simulink library "cstm_interfaces_lib"  (R2020a)
settings: Solver=VariableStepAuto  StartTime=0.0  StopTime=10.0  RelTol=1e-3
settings Model: Creator=niekl  LastModifiedBy=niekl

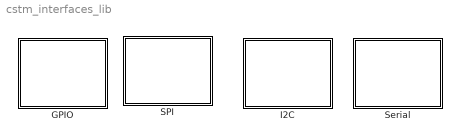
== system cstm_interfaces_lib ==
  GPIO : Subsystem
  I2C : Subsystem
  SPI : Subsystem
  Serial : Subsystem

== system cstm_interfaces_lib/GPIO ==
  cstm_GPIO_read : Subsystem  SystemSampleTime=inf  mask{port=0, OutDataTypeStr=boolean, SampleTime=-1}
      mask prompts: port "GPIO chip number"; OutDataTypeStr "Simulink:blkprm_prompts:OUTPUT_UNIFIEDDATATYPE"; SampleTime "Simulink:blkprm_prompts:AllBlksSampleTime"
      mask TypeOptions OutDataTypeStr: Cast To Boolean/OutDataTypeStr
      mask TypeOptions SampleTime: Val/SampleTime
      mask DialogControl OutDataTypeStr Prompt: Output data type:
      mask DialogControl SampleTime Prompt: Sample time (-1 for inherited):
      mask Display:
      | disp('cstm GPIO Read')
      | port_label('output', 1, 'Value')
  cstm_GPIO_write : Subsystem  mask{port=0, OutDataTypeStr=Inherit: auto, SampleTime=-1}
      mask prompts: port "GPIO chip number"; OutDataTypeStr "Simulink:blkprm_prompts:UNIFIEDDATATYPE"; SampleTime "Simulink:blkprm_prompts:AllBlksSampleTime"
      mask TypeOptions OutDataTypeStr: Val/OutDataTypeStr
      mask TypeOptions SampleTime: Val/SampleTime
      mask DialogControl OutDataTypeStr Prompt: Data type:
      mask DialogControl SampleTime Prompt: Sample time (-1 for inherited):
      mask Display:
      | disp('cstm GPIO Write')
      | port_label('input', 1, 'Value')

== system cstm_interfaces_lib/I2C ==
  cstm_I2C_Read : Subsystem  mask{ADAPTERNUMBER=0, ADDRESS=0, BYTEORDERSTRING=BigEndian, ENABLEREG=on, SLAVEREG=0, OutDataTypeStr=uint8, MESSAGESIZE=1, SENDNACKSTRING=on, REMOVESTOPSTRING=on, OUTERROR=off, BYTEORDER=0, SENDREGISTER=1, SENDNACK=1, REMOVESTOP=1}
      mask prompts: ADAPTERNUMBER "Adapter number:"; ADDRESS "Slave address:"; BYTEORDERSTRING "Slave byte order:"; ENABLEREG "Enable register access"; SLAVEREG "Slave register address:"; OutDataTypeStr "Simulink:blkprm_prompts:OUTPUT_UNIFIEDDATATYPE"; MESSAGESIZE "Data size:"; SENDNACKSTRING "Send NACK at end of data transfer"; REMOVESTOPSTRING "Remove stop bit at the end of data transfer"; OUTERROR "Output error status"; BYTEORDER "byte order translate"; SENDREGISTER "slave register address translate"; SENDNACK "send nack translate"; REMOVESTOP "remove stop bit translate"
      mask init:
      | enab = get_param(gcb,'OUTERROR');
      | 
      | % Set the 'MaskVisibilities' property for each parameters
      | if strcmp(enab,'on')
      |     if strcmp(get_param([gcb '/ErrorMessage'],'BlockType'), 'Display')
      |         replace_block(gcb, 'FollowLinks', 'on', 'Name', 'ErrorMessage', 'Outport', 'noprompt')
      |     end
      | else
      |     if strcmp(get_param([gcb '/ErrorMessage'],'BlockType'), 'Outport')
      |         replace_block(gcb, 'FollowLinks', 'on', 'Name', 'ErrorMessage', 'Display', 'noprompt')
      |     end
      | end
      mask TypeOptions BYTEORDERSTRING: BigEndian | LittleEndian
      mask Callback BYTEORDERSTRING:
      | if(strcmp(get_param(gcb,'BYTEORDERSTRING'),'BigEndian'))
      |     set_param(gcb, 'BYTEORDER', '0');
      | else
      |     set_param(gcb, 'BYTEORDER', '1');
      | end
      mask Callback ENABLEREG:
      | % Control parameter visiblity
      | 
      | % unchecked = 'off'
      | % checked = 'on'
      | enab = get_param(gcb,'ENABLEREG');
      | 
      | % Set the 'MaskVisibilities' property for each parameters
      | if strcmp(enab,'on')
      |     set_param(gcb, 'SENDREGISTER', '1');
      |     set_param(gcb,'MaskVisibilities',{'on','on','on','on','on','on','on','off','off','on','off','off','off','off'});
      | else
      |     set_param(gcb, 'SENDREGISTER', '0');
      |     set_param(gcb,'MaskVisibilities',{'on','on','on','on','off','on','on','on','on','on','off','off','off','off'});
      | end
      | 
      | % Note that the value of the bias is not handled here.
      | % See the Initialization tab
      mask TypeOptions OutDataTypeStr: Data Type Conversion/OutDataTypeStr
      mask Callback SENDNACKSTRING:
      | if(strcmp(get_param(gcb,'SENDNACKSTRING'),'off'))
      |     set_param(gcb, 'SENDNACK', '0');
      | else
      |     set_param(gcb, 'SENDNACK', '1');
      | end
      mask Callback REMOVESTOPSTRING:
      | if(strcmp(get_param(gcb,'REMOVESTOPSTRING'),'off'))
      |     set_param(gcb, 'REMOVESTOP', '0');
      | else
      |     set_param(gcb, 'REMOVESTOP', '1');
      | end
      mask DialogControl OutDataTypeStr Prompt: Output data type:
      mask DialogControl Container3 Prompt: hidden parameters for translation
      mask Display:
      | disp('cstm I2C Write')
      | port_label('output', 1, 'Message out')
      | 
      | if strcmp(get_param(gcb,'OUTERROR'),'on')
      |     port_label('output', 2, 'Error out')
      | end
  cstm_I2C_Write : Subsystem  mask{ADAPTERNUMBER=0, ADDRESS=0, BYTEORDERSTRING=BigEndian, ENABLEREG=on, SLAVEREG=0, SENDNACKSTRING=off, REMOVESTOPSTRING=off, OUTERROR=off, BYTEORDER=0, SENDREGISTER=1, SENDNACK=0, REMOVESTOP=0}
      mask prompts: ADAPTERNUMBER "Adapter number:"; ADDRESS "Slave address:"; BYTEORDERSTRING "Slave byte order:"; ENABLEREG "Enable register access"; SLAVEREG "Slave register address:"; SENDNACKSTRING "Send NACK at end of data transfer"; REMOVESTOPSTRING "Remove stop bit at the end of data transfer"; OUTERROR "Output error status"; BYTEORDER "byte order translate"; SENDREGISTER "slave register address translate"; SENDNACK "send nack translate"; REMOVESTOP "remove stop bit translate"
      mask init: same as cstm_interfaces_lib/I2C/cstm_I2C_Read
      mask TypeOptions BYTEORDERSTRING: BigEndian | LittleEndian
      mask Callback BYTEORDERSTRING:
      | if(strcmp(get_param(gcb,'BYTEORDERSTRING'),'BigEndian'))
      |     set_param(gcb, 'BYTEORDER', '0');
      | else
      |     set_param(gcb, 'BYTEORDER', '1');
      | end
      mask Callback ENABLEREG:
      | % Control parameter visiblity
      | 
      | % unchecked = 'off'
      | % checked = 'on'
      | enab = get_param(gcb,'ENABLEREG');
      | 
      | % Set the 'MaskVisibilities' property for each parameters
      | if strcmp(enab,'on')
      |     set_param(gcb, 'SENDREGISTER', '1');
      |     set_param(gcb,'MaskVisibilities',{'on','on','on','on','on','off','off','on','off','off','off','off'});
      | else
      |     set_param(gcb, 'SENDREGISTER', '0');
      |     set_param(gcb,'MaskVisibilities',{'on','on','on','on','off','on','on','on','off','off','off','off'});
      | end
      | 
      | % Note that the value of the bias is not handled here.
      | % See the Initialization tab
      mask Callback SENDNACKSTRING:
      | if(strcmp(get_param(gcb,'SENDNACKSTRING'),'off'))
      |     set_param(gcb, 'SENDNACK', '0');
      | else
      |     set_param(gcb, 'SENDNACK', '1');
      | end
      mask Callback REMOVESTOPSTRING:
      | if(strcmp(get_param(gcb,'REMOVESTOPSTRING'),'off'))
      |     set_param(gcb, 'REMOVESTOP', '0');
      | else
      |     set_param(gcb, 'REMOVESTOP', '1');
      | end
      mask DialogControl Container3 Prompt: hidden parameters for translation
      mask Display:
      | disp('cstm I2C Write')
      | port_label('input', 1, 'Message in')
      | 
      | if strcmp(get_param(gcb,'OUTERROR'),'on')
      |     port_label('output', 1, 'ErrorOut')
      | end

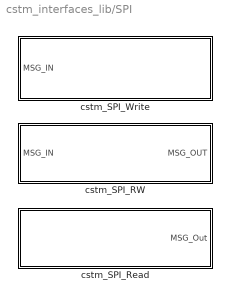
== system cstm_interfaces_lib/SPI ==
  cstm_SPI_RW : Subsystem  mask{Device=0, SlaveSelect=0, SelectedMode=0, RegisterAddress=0, DataLength=1, OutDataTypeStr_in=int8, OutDataTypeStr_out=int8, Sample=-1}
      mask prompts: Device "SPI device:"; SlaveSelect "SPI Slave Select:"; SelectedMode "Mode (Clock polarity and phase):"; RegisterAddress "Register address (-1 for none):"; DataLength "Data length (excluding register):"; OutDataTypeStr_in "Input data type:"; OutDataTypeStr_out "Simulink:blkprm_prompts:OUTPUT_UNIFIEDDATATYPE"; Sample "Sample time (-1 for inherited):"
      mask TypeOptions SelectedMode: 0 | 1 | 2 | 3
      mask DialogControl Control2 Prompt: Mode flag expects a value from 0 to 3: 1 sets phase flag, 2 sets clock polarity flag, and 3 sets both.
      mask DialogControl Control3 Prompt: Data can be read from a register. If this is not desired, set the Register address to -1.
      mask DialogControl Control4 Prompt: Data length expects a positive integer representing the amount of bytes to read. This number is the amount excluding the register address
      mask DialogControl Control6 Prompt: Input data expects a [Nx1] array
      mask DialogControl Control5 Prompt: Output data is a [Nx1] array
      mask DialogControl OutDataTypeStr_out Prompt: Output data type:
      mask Display:
      | disp('cstm SPI Write')
      | port_label('input', 1, 'MessageIn')
      | port_label('output', 1, 'MessageOut')
  cstm_SPI_Read : Subsystem  mask{Device=0, SlaveSelect=0, SelectedMode=0, RegisterAddress=0, DataLength=1, OutDataTypeStr_out=uint8, Sample=-1}
      mask prompts: Device "SPI device:"; SlaveSelect "SPI Slave Select:"; SelectedMode "Mode (Clock polarity and phase):"; RegisterAddress "Register address (-1 for none):"; DataLength "Data length (excluding register):"; OutDataTypeStr_out "Simulink:blkprm_prompts:OUTPUT_UNIFIEDDATATYPE"; Sample "Sample time (-1 for inherited):"
      mask TypeOptions SelectedMode: 0 | 1 | 2 | 3
      mask TypeOptions OutDataTypeStr_out: OutputCastTo/OutDataTypeStr
      mask DialogControl DescTextVar Prompt: Read and write data simultaniously using SPI with an optional register address
      mask DialogControl Control2 Prompt: Mode flag expects a value from 0 to 3: 1 sets phase flag, 2 sets clock polarity flag, and 3 sets both.
      mask DialogControl Control3 Prompt: Data can be read from a register. If this is not desired, set the Register address to -1.
      mask DialogControl Control4 Prompt: Data length expects a positive integer representing the amount of bytes to read and write. This number is the amount excluding the register address
      mask DialogControl Control5 Prompt: Output data is a [Nx1] array
      mask DialogControl OutDataTypeStr_out Prompt: Output data type:
      mask Display:
      | disp('cstm SPI Write')
      | port_label('output', 1, 'MessageOut')
  cstm_SPI_Write : Subsystem  mask{Device=0, SlaveSelect=0, SelectedMode=0, RegisterAddress=0, OutDataTypeStr_out=Inherit: auto, Sample=-1}
      mask prompts: Device "SPI device:"; SlaveSelect "SPI Slave Select:"; SelectedMode "Mode (Clock polarity and phase):"; RegisterAddress "Register address (-1 for none):"; OutDataTypeStr_out "Input data type:"; Sample "Sample time (-1 for inherited):"
      mask TypeOptions SelectedMode: 0 | 1 | 2 | 3
      mask TypeOptions OutDataTypeStr_out: MSG_IN/OutDataTypeStr
      mask DialogControl DescTextVar Prompt: Write data using SPI
      mask DialogControl Control4 Prompt: Mode flag expects a value from 0 to 3: 1 sets phase flag, 2 sets clock polarity flag, and 3 sets both.
      mask DialogControl Control2 Prompt: Data can be written to a register. If this is not desired, set the Register address to -1.
      mask DialogControl Control3 Prompt: Input data expects a [Nx1] array
      mask Display:
      | disp('cstm SPI Write')
      | port_label('input', 1, 'MessageIn')

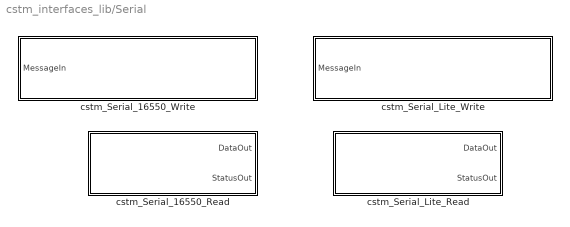
== system cstm_interfaces_lib/Serial ==
  cstm_Serial_16550_Read : Subsystem  mask{PORT=0, BAUDRATE=115200, PARITYSTRING=None, STOPBITS=1, DATALENGTH=1, DATATYPE=int8, SampleTime=-1, BAUDRATESS=0, PARITY=0}
      mask prompts: PORT "Port (ttyS<x>):"; BAUDRATE "Baudrate (in bits/s):"; PARITYSTRING "Parity:"; STOPBITS "Stop bits"; DATALENGTH "Data length (N):"; DATATYPE "Output data type:"; SampleTime "Simulink:blkprm_prompts:AllBlksSampleTime"; BAUDRATESS "baudrate translate"; PARITY "parity translate"
      mask TypeOptions BAUDRATE: 0 | 50 | 75 | 110 | 134 | 150 | 200 | 300 | 600 | 1200 | 1800 | 2400 | 4800 | 9600 | 19200 | 38400 | 57600 | 115200 | 230400
      mask Callback BAUDRATE:
      | % baud = get_param(gcb, 'BAUDRATESTRING')
      | %
      | % switch(baud)
      | %     case '0'
      | %         set_param(gcb,'BAUDRATE','0');
      | %     case '50'
      | %         set_param(gcb,'BAUDRATE','50');
      | %     case '75'
      | %         set_param(gcb,'BAUDRATE','75');
      | %     case '110'
      | %         set_param(gcb,'BAUDRATE','110');
      | %     case '134'
      | %         set_param(gcb,'BAUDRATE','134');
      | %     case '150'
      | %         set_param(gcb,'BAUDRATE','150');
      | %     case '200'
      | %         set_param(gcb,'BAUDRATE','200');
      | %     case '300'
      | %         set_param(gcb,'BAUDRATE','300');
      | %     case '600'
      | %         set_param(gcb,'BAUDRATE','600');
      | %     case '1200'
      | %         set_param(gcb,'BAUDRATE','1200');
      | %     case '0'
      | %         set_param(gcb,'BAUDRATE','1800');
      | %     case '0'
      | %         set_param(gcb,'BAUDRATE','2400');
      | %     case '0'
      | %         set_param(gcb,'BAUDRATE','4800');
      | %     case '0'
      | %         set_param(gcb,'BAUDRATE','9600');
      | %     case '0'
      | %         set_param(gcb,'BAUDRATE','19200');
      | %     case '0'
      | %         set_param(gcb,'BAUDRATE','38400');
      | %     case '0'
      | %         set_param(gcb,'BAUDRATE','57600');
      | %     case '0'
      | %         set_param(gcb,'BAUDRATE','115200');
      | %     case '0'
      | %         set_param(gcb,'BAUDRATE','230400');
      | % end
      mask TypeOptions PARITYSTRING: None | Even | Odd
      mask Callback PARITYSTRING:
      | if(strcmp(get_param(gcb, 'PARITYSTRING'),'none'))
      |     set_param(gcb,'PARITY','0');
      | end
      | if(strcmp(get_param(gcb, 'PARITYSTRING'),'Even'))
      |     set_param(gcb,'PARITY','1');
      | end
      | if(strcmp(get_param(gcb, 'PARITYSTRING'),'Odd'))
      |     set_param(gcb,'PARITY','2');
      | end
      mask TypeOptions STOPBITS: 1 | 2
      mask Callback DATALENGTH:
      | %ph = get_param(gcb,'PortHandles');
      | %length = get_param(gcb, 'DATALENGTH');
      | %set_param([gcb '/DataOut'],'CompiledPortWidths',length);
      mask TypeOptions SampleTime: Data Type Conversion/SampleTime
      mask DialogControl Control2 Prompt: The output: "Message out" is an array of size [Nx1]. Any data presented to UART16550 will be received, upto N bytes (max 256).
      mask DialogControl Control3 Prompt: The output: "Status out" is a [1x1] variable with the amount of read bytes.
      mask DialogControl SampleTime Prompt: Sample time (-1 for inherited):
      mask DialogControl Container3 Prompt: hidden
      mask Display:
      | disp('cstm Serial 16550 Read')
      | port_label('output', 1, 'Message out')
      | port_label('output', 2, 'Status out')
  cstm_Serial_16550_Write : Subsystem  mask{PORT=0, BAUDRATE=0, PARITYSTRING=None, STOPBITS=1, PARITY=0}
      mask prompts: PORT "Port (ttyS<x>):"; BAUDRATE "Baudrate (in bits/s):"; PARITYSTRING "Parity:"; STOPBITS "Stop bits"; PARITY "parity translate"
      mask TypeOptions BAUDRATE: 0 | 50 | 75 | 110 | 134 | 150 | 200 | 300 | 600 | 1200 | 1800 | 2400 | 4800 | 9600 | 19200 | 38400 | 57600 | 115200 | 230400
      mask TypeOptions PARITYSTRING: None | Even | Odd
      mask Callback PARITYSTRING:
      | if(strcmp(get_param(gcb, 'PARITYSTRING'),'none'))
      |     set_param(gcb,'PARITY','0');
      | end
      | if(strcmp(get_param(gcb, 'PARITYSTRING'),'Even'))
      |     set_param(gcb,'PARITY','1');
      | end
      | if(strcmp(get_param(gcb, 'PARITYSTRING'),'Odd'))
      |     set_param(gcb,'PARITY','2');
      | end
      mask TypeOptions STOPBITS: 1 | 2
      mask DialogControl Control2 Prompt: The input is an array of size [Nx1]. Any data presented to UART16550 will be transmitted.
      mask Display:
      | disp('cstm Serial 16550 Write')
      | port_label('input', 1, 'Message in')
  cstm_Serial_Lite_Read : Subsystem  mask{PORT=0, DATALENGTH=0, DATATYPE=int8, SampleTime=-1}
      mask prompts: PORT "Port (ttyUL<x>):"; DATALENGTH "Data length (N):"; DATATYPE "Output data type:"; SampleTime "Simulink:blkprm_prompts:AllBlksSampleTime"
      mask TypeOptions SampleTime: Data Type Conversion/SampleTime
      mask DialogControl DescTextVar Prompt: UARTlite Read accepts only the port as parameter, the device has been pre-configured and cannot be configured in the user space. Contact the SoC developer for details of the UARTlite device in use.
      mask DialogControl Control2 Prompt: The output: "Message out" is an array of size [Nx1]. Any data presented to UARTlite will be received, upto N bytes (max 256).
      mask DialogControl Control2_copy Prompt: The output: "Status out" is a [1x1] variable with the amount of read bytes.
      mask DialogControl SampleTime Prompt: Sample time (-1 for inherited):
      mask Display:
      | disp('cstm Serial Lite Read')
      | port_label('output', 1, 'Message out')
      | port_label('output', 2, 'Status out')
  cstm_Serial_Lite_Write : Subsystem  mask{PORT=0}
      mask prompts: PORT "Port (ttyUL<x>):"
      mask DialogControl DescTextVar Prompt: UARTlite Write accepts only the port as parameter, the device has been pre-configured and cannot be configured in the user space. Contact the SoC developer for details of the UARTlite device in use.
      mask DialogControl Control2 Prompt: The input is an array of size [Nx1]. Any data presented to UARTlite will be transmitted.
      mask Display:
      | disp('cstm Serial Lite Write')
      | port_label('input', 1, 'Message in')

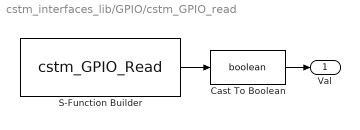
== system cstm_interfaces_lib/GPIO/cstm_GPIO_read ==
  Cast To Boolean : DataTypeConversion  OutDataTypeStr=boolean
  S-Function Builder : S-Function  InitFcn=try, set_param(gcb,'FunctionName','cstm_GPIO_Read'), end  FunctionName=cstm_GPIO_Read  Parameters=uint32(port)  SFunctionModules=cstm_GPIO_Read_wrapper  SFunctionDeploymentMode=off  EnableBusSupport=off  mask(S-Function Builder){}
      mask help: Simulink:masks:SFunctionBuilder_MD
      mask init:
      | val = [[.9  0.75 0.75 1 1 .9 .9 1]',[1 1 0.75 0.75 .9 .9 1 .9]'];try , sys = get_param(gcb,'SfunBuilderFcnName');if isempty(sys), sys = get_param(gcb,'FunctionName'); end,catch, sys = get_param(gcb,'FunctionName'); end
      settings: CopyFcn=set_param(gcbh,'LinkStatus','none')  PreSaveFcn=try, set_param(gcb,'FunctionName','cstm_GPIO_Read'), end  OpenFcn=sfunctionwizard(gcbh)
      mask Display: plot(val(:,1),val(:,2)),disp(sys), port_label('output',1,'Val')
  Val : Outport  OutDataTypeStr=boolean  SampleTime=SampleTime
  wires:
  S-Function Builder/1 -> Cast To Boolean/1
  Cast To Boolean/1 -> Val/1

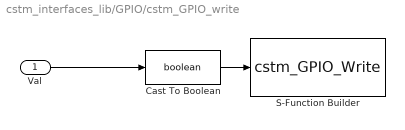
== system cstm_interfaces_lib/GPIO/cstm_GPIO_write ==
  Val : Inport  SampleTime=SampleTime
  Cast To Boolean : DataTypeConversion  OutDataTypeStr=boolean
  S-Function Builder : S-Function  InitFcn=try, set_param(gcb,'FunctionName','cstm_GPIO_Write'), end  FunctionName=cstm_GPIO_Write  Parameters=uint32(port)  SFunctionModules=cstm_GPIO_Write_wrapper  SFunctionDeploymentMode=off  EnableBusSupport=off  mask(S-Function Builder){}
      mask help: Simulink:masks:SFunctionBuilder_MD
      mask init: same as cstm_interfaces_lib/GPIO/cstm_GPIO_read/S-Function Builder
      settings: CopyFcn=set_param(gcbh,'LinkStatus','none')  PreSaveFcn=try, set_param(gcb,'FunctionName','cstm_GPIO_Write'), end  OpenFcn=sfunctionwizard(gcbh)
      mask Display: plot(val(:,1),val(:,2)),disp(sys), port_label('input',1,'Val')
  wires:
  Val/1 -> Cast To Boolean/1
  Cast To Boolean/1 -> S-Function Builder/1

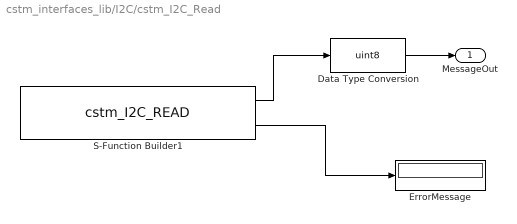
== system cstm_interfaces_lib/I2C/cstm_I2C_Read ==
  Data Type Conversion : DataTypeConversion  OutDataTypeStr=uint8
  ErrorMessage : Display
  S-Function Builder1 : S-Function  InitFcn=try, set_param(gcb,'FunctionName','cstm_I2C_READ'), end  FunctionName=cstm_I2C_READ  Parameters=uint8(ADDRESS),uint8(ADAPTERNUMBER),uint8(BYTEORDER),uint8(MESSAGESIZE),uint8(SENDREGISTER),uint8(SLAVEREG),uint8(SENDNACK),uint8(REMOVESTOP)  SFunctionModules=cstm_I2C_READ_wrapper  SFunctionDeploymentMode=off  EnableBusSupport=off  mask(S-Function Builder){}
      mask help: Simulink:masks:SFunctionBuilder_MD
      mask init: same as cstm_interfaces_lib/GPIO/cstm_GPIO_read/S-Function Builder
      settings: CopyFcn=set_param(gcbh,'LinkStatus','none')  PreSaveFcn=try, set_param(gcb,'FunctionName','cstm_I2C_READ'), end  OpenFcn=sfunctionwizard(gcbh)
      mask Display: plot(val(:,1),val(:,2)),disp(sys), port_label('output',1,'OutputMessage'), port_label('output',2,'ErrorStatus')
  MessageOut : Outport  PortDimensions=MESSAGESIZE
  wires:
  S-Function Builder1/2 -> ErrorMessage/1
  Data Type Conversion/1 -> MessageOut/1
  S-Function Builder1/1 -> Data Type Conversion/1

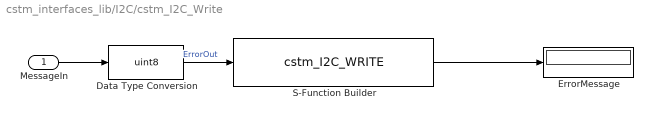
== system cstm_interfaces_lib/I2C/cstm_I2C_Write ==
  MessageIn : Inport
  Data Type Conversion : DataTypeConversion  OutDataTypeStr=uint8
  ErrorMessage : Display
  S-Function Builder : S-Function  InitFcn=try, set_param(gcb,'FunctionName','cstm_I2C_WRITE'), end  FunctionName=cstm_I2C_WRITE  Parameters=uint8(ADDRESS),uint8(ADAPTERNUMBER),uint8(BYTEORDER),uint8(SENDREGISTER),uint8(SLAVEREG),uint8(SENDNACK),uint8(REMOVESTOP)  SFunctionModules=cstm_I2C_WRITE_wrapper  SFunctionDeploymentMode=off  EnableBusSupport=off  mask(S-Function Builder){}
      mask help: Simulink:masks:SFunctionBuilder_MD
      mask init: same as cstm_interfaces_lib/GPIO/cstm_GPIO_read/S-Function Builder
      settings: CopyFcn=set_param(gcbh,'LinkStatus','none')  PreSaveFcn=try, set_param(gcb,'FunctionName','cstm_I2C_WRITE'), end  OpenFcn=sfunctionwizard(gcbh)
      mask Display: plot(val(:,1),val(:,2)),disp(sys), port_label('input',1,'InputMessage'), port_label('output',1,'ErrorStatus')
  wires:
  MessageIn/1 -> Data Type Conversion/1
  Data Type Conversion/1 -> S-Function Builder/1  "ErrorOut"
  S-Function Builder/1 -> ErrorMessage/1

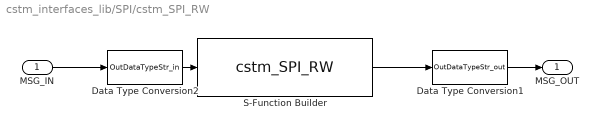
== system cstm_interfaces_lib/SPI/cstm_SPI_RW ==
  MSG_IN : Inport  PortDimensions=DataLength  SampleTime=Sample
  Data Type Conversion1 : DataTypeConversion  OutDataTypeStr=OutDataTypeStr_out
  Data Type Conversion2 : DataTypeConversion  OutDataTypeStr=OutDataTypeStr_in
  S-Function Builder : S-Function  InitFcn=try, set_param(gcb,'FunctionName','cstm_SPI_RW'), end  FunctionName=cstm_SPI_RW  Parameters=uint32(Device),uint32(SlaveSelect),int32(RegisterAddress),int32(SelectedMode),uint32(DataLength)  SFunctionModules=cstm_SPI_RW_wrapper  SFunctionDeploymentMode=off  EnableBusSupport=off  mask(S-Function Builder){}
      mask help: Simulink:masks:SFunctionBuilder_MD
      mask init: same as cstm_interfaces_lib/GPIO/cstm_GPIO_read/S-Function Builder
      settings: CopyFcn=set_param(gcbh,'LinkStatus','none')  PreSaveFcn=try, set_param(gcb,'FunctionName','cstm_SPI_RW'), end  OpenFcn=sfunctionwizard(gcbh)
      mask Display: plot(val(:,1),val(:,2)),disp(sys), port_label('input',1,'InputByte'), port_label('output',1,'OutputByte')
  MSG_OUT : Outport  PortDimensions=DataLength  SampleTime=Sample
  wires:
  Data Type Conversion1/1 -> MSG_OUT/1
  S-Function Builder/1 -> Data Type Conversion1/1
  Data Type Conversion2/1 -> S-Function Builder/1
  MSG_IN/1 -> Data Type Conversion2/1

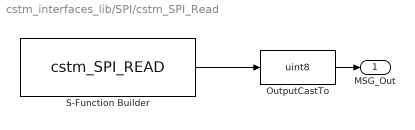
== system cstm_interfaces_lib/SPI/cstm_SPI_Read ==
  OutputCastTo : DataTypeConversion  OutDataTypeStr=uint8
  S-Function Builder : S-Function  InitFcn=try, set_param(gcb,'FunctionName','cstm_SPI_READ'), end  FunctionName=cstm_SPI_READ  Parameters=uint32(Device),uint32(SlaveSelect),int32(RegisterAddress),int32(SelectedMode),uint32(DataLength)  SFunctionModules=cstm_SPI_READ_wrapper  SFunctionDeploymentMode=off  EnableBusSupport=off  mask(S-Function Builder){}
      mask help: Simulink:masks:SFunctionBuilder_MD
      mask init: same as cstm_interfaces_lib/GPIO/cstm_GPIO_read/S-Function Builder
      settings: CopyFcn=set_param(gcbh,'LinkStatus','none')  PreSaveFcn=try, set_param(gcb,'FunctionName','cstm_SPI_READ'), end  OpenFcn=sfunctionwizard(gcbh)
      mask Display: plot(val(:,1),val(:,2)),disp(sys), port_label('output',1,'OutputByte')
  MSG_Out : Outport  PortDimensions=DataLength  SampleTime=Sample
  wires:
  OutputCastTo/1 -> MSG_Out/1
  S-Function Builder/1 -> OutputCastTo/1

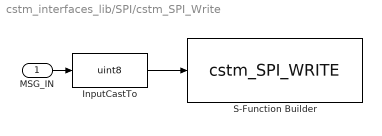
== system cstm_interfaces_lib/SPI/cstm_SPI_Write ==
  MSG_IN : Inport  SampleTime=Sample
  InputCastTo : DataTypeConversion  OutDataTypeStr=uint8
  S-Function Builder : S-Function  InitFcn=try, set_param(gcb,'FunctionName','cstm_SPI_WRITE'), end  FunctionName=cstm_SPI_WRITE  Parameters=uint32(Device),uint32(SlaveSelect),int32(RegisterAddress),int32(SelectedMode)  SFunctionModules=cstm_SPI_WRITE_wrapper  SFunctionDeploymentMode=off  EnableBusSupport=off  mask(S-Function Builder){}
      mask help: Simulink:masks:SFunctionBuilder_MD
      mask init: same as cstm_interfaces_lib/GPIO/cstm_GPIO_read/S-Function Builder
      settings: CopyFcn=set_param(gcbh,'LinkStatus','none')  PreSaveFcn=try, set_param(gcb,'FunctionName','cstm_SPI_WRITE'), end  OpenFcn=sfunctionwizard(gcbh)
      mask Display: plot(val(:,1),val(:,2)),disp(sys), port_label('input',1,'InputByte')
  wires:
  MSG_IN/1 -> InputCastTo/1
  InputCastTo/1 -> S-Function Builder/1

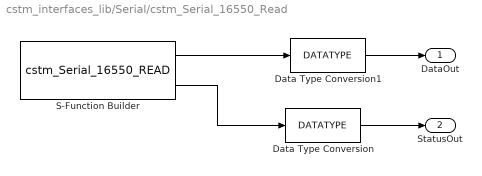
== system cstm_interfaces_lib/Serial/cstm_Serial_16550_Read ==
  Data Type Conversion : DataTypeConversion  OutDataTypeStr=DATATYPE  SampleTime=SampleTime
  Data Type Conversion1 : DataTypeConversion  OutDataTypeStr=DATATYPE  SampleTime=SampleTime
  S-Function Builder : S-Function  InitFcn=try, set_param(gcb,'FunctionName','cstm_Serial_16550_READ'), end  FunctionName=cstm_Serial_16550_READ  Parameters=uint32(PORT),uint32(BAUDRATE),uint32(PARITY),uint32(STOPBITS),uint32(DATALENGTH)  SFunctionModules=cstm_Serial_16550_READ_wrapper  SFunctionDeploymentMode=off  EnableBusSupport=off  mask(S-Function Builder){}
      mask help: Simulink:masks:SFunctionBuilder_MD
      mask init: same as cstm_interfaces_lib/GPIO/cstm_GPIO_read/S-Function Builder
      settings: CopyFcn=set_param(gcbh,'LinkStatus','none')  PreSaveFcn=try, set_param(gcb,'FunctionName','cstm_Serial_16550_READ'), end  OpenFcn=sfunctionwizard(gcbh)
      mask Display: plot(val(:,1),val(:,2)),disp(sys), port_label('output',1,'Data'), port_label('output',2,'Status')
  DataOut : Outport  PortDimensions=DATALENGTH
  StatusOut : Outport  Port=2
  wires:
  S-Function Builder/2 -> Data Type Conversion/1
  Data Type Conversion/1 -> StatusOut/1
  Data Type Conversion1/1 -> DataOut/1
  S-Function Builder/1 -> Data Type Conversion1/1

== system cstm_interfaces_lib/Serial/cstm_Serial_16550_Write ==
  MessageIn : Inport
  Data Type Conversion1 : DataTypeConversion  OutDataTypeStr=uint8
  S-Function Builder1 : S-Function  InitFcn=try, set_param(gcb,'FunctionName','cstm_Serial_16550_Write'), end  FunctionName=cstm_Serial_16550_Write  Parameters=uint32(PORT),uint32(BAUDRATE),uint32(PARITY),uint32(STOPBITS)  SFunctionModules=cstm_Serial_16550_Write_wrapper  SFunctionDeploymentMode=off  EnableBusSupport=off  mask(S-Function Builder){}
      mask help: Simulink:masks:SFunctionBuilder_MD
      mask init: same as cstm_interfaces_lib/GPIO/cstm_GPIO_read/S-Function Builder
      settings: CopyFcn=set_param(gcbh,'LinkStatus','none')  PreSaveFcn=try, set_param(gcb,'FunctionName','cstm_Serial_16550_Write'), end  OpenFcn=sfunctionwizard(gcbh)
      mask Display: plot(val(:,1),val(:,2)),disp(sys), port_label('input',1,'Data')
  wires:
  Data Type Conversion1/1 -> S-Function Builder1/1
  MessageIn/1 -> Data Type Conversion1/1

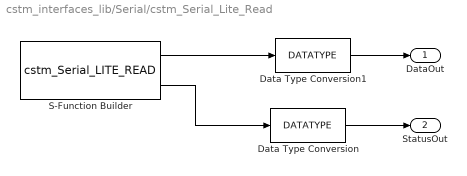
== system cstm_interfaces_lib/Serial/cstm_Serial_Lite_Read ==
  Data Type Conversion : DataTypeConversion  OutDataTypeStr=DATATYPE  SampleTime=SampleTime
  Data Type Conversion1 : DataTypeConversion  OutDataTypeStr=DATATYPE  SampleTime=SampleTime
  S-Function Builder : S-Function  InitFcn=try, set_param(gcb,'FunctionName','cstm_Serial_LITE_READ'), end  FunctionName=cstm_Serial_LITE_READ  Parameters=uint32(PORT),uint32(DATALENGTH)  SFunctionModules=cstm_Serial_LITE_READ_wrapper  SFunctionDeploymentMode=off  EnableBusSupport=off  mask(S-Function Builder){}
      mask help: Simulink:masks:SFunctionBuilder_MD
      mask init: same as cstm_interfaces_lib/GPIO/cstm_GPIO_read/S-Function Builder
      settings: CopyFcn=set_param(gcbh,'LinkStatus','none')  PreSaveFcn=try, set_param(gcb,'FunctionName','cstm_Serial_LITE_READ'), end  OpenFcn=sfunctionwizard(gcbh)
      mask Display: plot(val(:,1),val(:,2)),disp(sys), port_label('output',1,'Data'), port_label('output',2,'Status')
  DataOut : Outport  PortDimensions=DATALENGTH
  StatusOut : Outport  Port=2
  wires:
  Data Type Conversion/1 -> StatusOut/1
  S-Function Builder/2 -> Data Type Conversion/1
  S-Function Builder/1 -> Data Type Conversion1/1
  Data Type Conversion1/1 -> DataOut/1

== system cstm_interfaces_lib/Serial/cstm_Serial_Lite_Write ==
  MessageIn : Inport
  Data Type Conversion1 : DataTypeConversion  OutDataTypeStr=uint8
  S-Function Builder1 : S-Function  InitFcn=try, set_param(gcb,'FunctionName','cstm_Serial_LITE_Write'), end  FunctionName=cstm_Serial_LITE_Write  Parameters=uint32(PORT)  SFunctionModules=cstm_Serial_LITE_Write_wrapper  SFunctionDeploymentMode=off  EnableBusSupport=off  mask(S-Function Builder){}
      mask help: Simulink:masks:SFunctionBuilder_MD
      mask init: same as cstm_interfaces_lib/GPIO/cstm_GPIO_read/S-Function Builder
      settings: CopyFcn=set_param(gcbh,'LinkStatus','none')  PreSaveFcn=try, set_param(gcb,'FunctionName','cstm_Serial_LITE_Write'), end  OpenFcn=sfunctionwizard(gcbh)
      mask Display: plot(val(:,1),val(:,2)),disp(sys), port_label('input',1,'Data')
  wires:
  MessageIn/1 -> Data Type Conversion1/1
  Data Type Conversion1/1 -> S-Function Builder1/1
